simulink model "Simulink_motor_x_est_int_obs"  (R2018a)
settings: Solver=VariableStepAuto  StartTime=0.0  StopTime=10  RelTol=1e-3
undefined symbols (not defined in the file): A_X, A_Y, Ax_d, Ay_d, B_X, B_Y, Bx_d, By_d, C_X, C_Y, Cx_d, Cy_d, DiscIntNeverNeededParam, dt, Kix_d, Kix_I, Kiy_d, Kiy_I, Lx, Ly
settings Model: Creator=DELL  LastModifiedBy=DELL
settings DataIOCC: ReturnWorkspaceOutputs=on
settings SFSimCC: SimUseLocalCustomCode=on
settings RTWCC: RTWUseLocalCustomCode=on

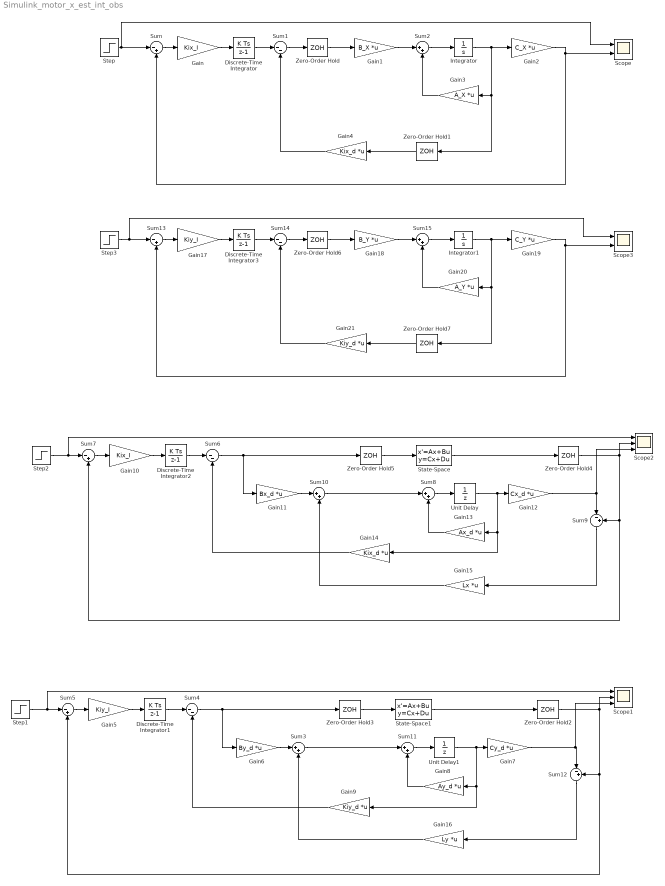
== system Simulink_motor_x_est_int_obs ==
  Discrete-Time Integrator{,1..3} (4 alike) : DiscreteIntegrator  SampleTime=dt  ICPrevOutput=DiscIntNeverNeededParam  ICPrevScaledInput=DiscIntNeverNeededParam
  Gain : Gain  Gain=Kix_I
  Gain1 : Gain  Gain=B_X  Multiplication=Matrix(K*u)
  Gain10 : Gain  Gain=Kix_I
  Gain11 : Gain  Gain=Bx_d  Multiplication=Matrix(K*u)
  Gain12 : Gain  Gain=Cx_d  Multiplication=Matrix(K*u)
  Gain13 : Gain  Gain=Ax_d  Multiplication=Matrix(K*u)
  Gain14 : Gain  Gain=Kix_d  Multiplication=Matrix(K*u)
  Gain15 : Gain  Gain=Lx  Multiplication=Matrix(K*u)
  Gain16 : Gain  Gain=Ly  Multiplication=Matrix(K*u)
  Gain17 : Gain  Gain=Kiy_I
  Gain18 : Gain  Gain=B_Y  Multiplication=Matrix(K*u)
  Gain19 : Gain  Gain=C_Y  Multiplication=Matrix(K*u)
  Gain2 : Gain  Gain=C_X  Multiplication=Matrix(K*u)
  Gain20 : Gain  Gain=A_Y  Multiplication=Matrix(K*u)
  Gain21 : Gain  Gain=Kiy_d  Multiplication=Matrix(K*u)
  Gain3 : Gain  Gain=A_X  Multiplication=Matrix(K*u)
  Gain4 : Gain  Gain=Kix_d  Multiplication=Matrix(K*u)
  Gain5 : Gain  Gain=Kiy_I
  Gain6 : Gain  Gain=By_d  Multiplication=Matrix(K*u)
  Gain7 : Gain  Gain=Cy_d  Multiplication=Matrix(K*u)
  Gain8 : Gain  Gain=Ay_d  Multiplication=Matrix(K*u)
  Gain9 : Gain  Gain=Kiy_d  Multiplication=Matrix(K*u)
  Integrator : Integrator
  Integrator1 : Integrator
  Scope : Scope  NumInputPorts=2
  Scope1 : Scope  NumInputPorts=3
  Scope2 : Scope  NumInputPorts=3
  Scope3 : Scope  NumInputPorts=2
  State-Space : StateSpace  A=A_X  B=B_X  C=C_X  D=0  InitialCondition=0
  State-Space1 : StateSpace  A=A_Y  B=B_Y  C=C_Y  D=0  InitialCondition=0
  Step{,1..3} (4 alike) : Step  Time=2  SampleTime=dt
  Sum{,5,7,9,12..13} (6 alike) : Sum  Inputs=|-+
  Sum{1,4,6,14} (4 alike) : Sum  Inputs=|--
  Sum{2..3,8,10..11,15} (6 alike) : Sum  Inputs=|++
  Unit Delay : UnitDelay  SampleTime=-1  HasFrameUpgradeWarning=on
  Unit Delay1 : UnitDelay  SampleTime=-1  HasFrameUpgradeWarning=on
  Zero-Order Hold{,1..7} (8 alike) : ZeroOrderHold  SampleTime=dt
  wires:
  Sum/1 -> Gain/1
  Gain/1 -> Discrete-Time Integrator/1
  Discrete-Time Integrator/1 -> Sum1/1
  Sum1/1 -> Zero-Order Hold/1
  Zero-Order Hold/1 -> Gain1/1
  Gain1/1 -> Sum2/1
  Sum2/1 -> Integrator/1
  Integrator/1 -> Gain3/1, Zero-Order Hold1/1, Gain2/1
  Gain3/1 -> Sum2/2
  Zero-Order Hold1/1 -> Gain4/1
  Gain4/1 -> Sum1/2
  Gain2/1 -> Scope/2, Sum/2
  Sum6/1 -> Gain11/1, Zero-Order Hold5/1
  Gain10/1 -> Discrete-Time Integrator2/1
  Step2/1 -> Scope2/1, Sum7/1
  Discrete-Time Integrator2/1 -> Sum6/1
  Sum7/1 -> Gain10/1
  Gain13/1 -> Sum8/2
  Sum10/1 -> Sum8/1
  Sum8/1 -> Unit Delay/1
  Unit Delay/1 -> Gain14/1, Gain13/1, Gain12/1
  Gain12/1 -> Scope2/3, Sum9/1
  Gain14/1 -> Sum6/2
  Gain15/1 -> Sum10/2
  Gain11/1 -> Sum10/1
  Sum9/1 -> Gain15/1
  Zero-Order Hold5/1 -> State-Space/1
  Zero-Order Hold4/1 -> Sum9/2, Sum7/2, Scope2/2
  State-Space/1 -> Zero-Order Hold4/1
  Unit Delay1/1 -> Gain9/1, Gain8/1, Gain7/1
  Gain7/1 -> Scope1/3, Sum12/1
  Gain16/1 -> Sum3/2
  Gain6/1 -> Sum3/1
  Gain8/1 -> Sum11/2
  Gain9/1 -> Sum4/2
  Sum11/1 -> Unit Delay1/1
  Sum5/1 -> Gain5/1
  Sum3/1 -> Sum11/1
  Sum12/1 -> Gain16/1
  Step1/1 -> Scope1/1, Sum5/1
  Gain5/1 -> Discrete-Time Integrator1/1
  Sum4/1 -> Gain6/1, Zero-Order Hold3/1
  State-Space1/1 -> Zero-Order Hold2/1
  Discrete-Time Integrator1/1 -> Sum4/1
  Zero-Order Hold2/1 -> Sum12/2, Sum5/2, Scope1/2
  Zero-Order Hold3/1 -> State-Space1/1
  Gain18/1 -> Sum15/1
  Step3/1 -> Scope3/1, Sum13/1
  Zero-Order Hold7/1 -> Gain21/1
  Sum14/1 -> Zero-Order Hold6/1
  Integrator1/1 -> Gain20/1, Zero-Order Hold7/1, Gain19/1
  Gain20/1 -> Sum15/2
  Sum15/1 -> Integrator1/1
  Discrete-Time Integrator3/1 -> Sum14/1
  Gain21/1 -> Sum14/2
  Sum13/1 -> Gain17/1
  Zero-Order Hold6/1 -> Gain18/1
  Gain19/1 -> Scope3/2, Sum13/2
  Gain17/1 -> Discrete-Time Integrator3/1
  Step/1 -> Scope/1, Sum/1
